simulink model "Engine"  (Simulink 9.3)
settings: Solver=ode23tb  StartTime=0.0  StopTime=50  FixedStep=0.001  EnableMultiTasking=on
values from neighbouring files (symbols this model uses):
  toggle_paf = toggle(2)    [RunEngine.m]
  toggle_vol = toggle(3)    [RunEngine.m]
  toggle_Waf = toggle(4)    [RunEngine.m]
  toggle_Wc = toggle(5)    [RunEngine.m]
  toggle_Wic = toggle(6)    [RunEngine.m]
  toggle_Wth = toggle(7)    [RunEngine.m]
  toggle_xth = toggle(8)    [RunEngine.m]
  toggle_ypic = toggle(9)    [RunEngine.m]
  toggle_ypim = toggle(10)    [RunEngine.m]
  toggle_yTic = toggle(11)    [RunEngine.m]
  toggle_yWaf = toggle(12)    [RunEngine.m]
undefined symbols (not defined in the file or in its folder): a0, a1, a2, dP_thrREF, KpThr, KpWg, n_r, Newton, r_c, Raphson, T_z, TC_ENGINE, TiThr, TiWg
libraries: simulink x3
(part 1 of 3)
settings Model: Creator=Mark Ng  LastModifiedBy=markng  ExtModeTrigMode=oneshot  ExtModeArmWhenConnect=off  ExtModeAutoUpdateStatusClock=off
settings SolverCC: MaxConsecutiveMinStep=100  ZeroCrossControl=EnableAll  SolverResetMethod=Robust
settings DataIOCC: SignalLoggingName=sigsOut
settings OptimizationCC: BooleanDataType=off  ExpressionDepthLimit=2147483647  InitFltsAndDblsToZero=on  SimCompilerOptimization=on
settings DebuggingCC: SaveWithParameterizedLinksMsg=none  SignalResolutionControl=TryResolveAllWithWarning  MaxConsecutiveZCsMsg=none  MultiTaskDSMMsg=warning  MultiTaskCondExecSysMsg=none  StateNameClashWarn=warning  PregeneratedLibrarySubsystemCodeDiagnostic=none
settings HardwareCC: TargetBitPerLong=64  TargetBitPerPointer=64  TargetBitPerSizeT=64  TargetBitPerPtrDiffT=64  TargetLongLongMode=on  TargetIntDivRoundTo=Zero  TargetEndianess=LittleEndian  TargetWordSize=64  TargetHWDeviceType=MATLAB Host  ProdEqTarget=off
settings GRTTargetCC: TargetFcnLib=ansi_tfl_tmw.mat  CompOptLevelCompliant=off  GeneratePreprocessorConditionals=Disable all

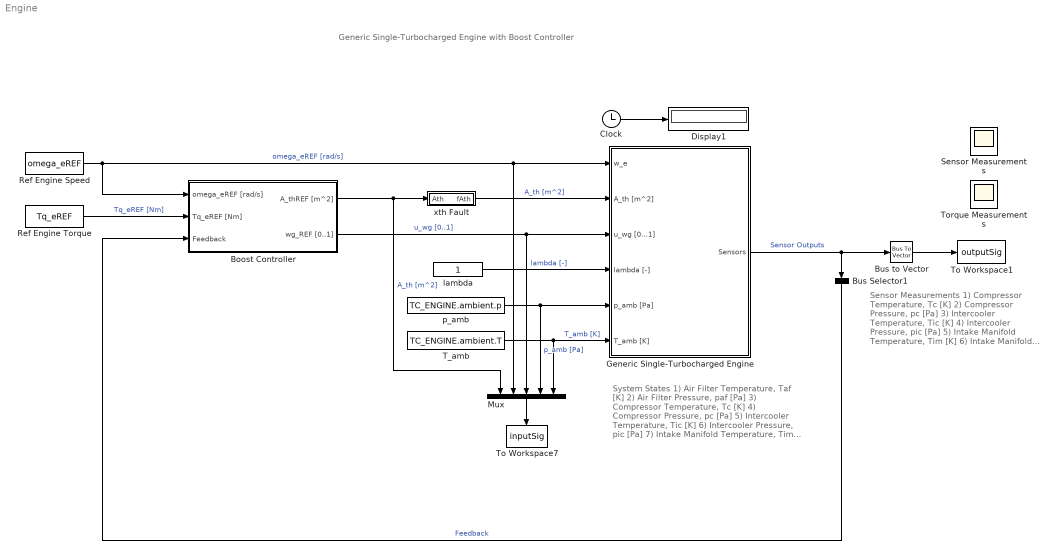
== system Engine ==
  note: Sensor Measurements
      |
      | 1) Compressor Temperature, Tc [K]
      | 2) Compressor Pressure, pc [Pa]
      | 3) Intercooler Temperature, Tic [K]
      | 4) Intercooler Pressure, pic [Pa]
      | 5) Intake Manifold Temperature, Tim [K]
      | 6) Intake Manifold Pressure, pim [Pa]
      | 7) Air Filter Mass Flow, Waf [kg/s]
      | 8) Engine Torque, Tq_e [Nm]
      | 9) Exhaust Manifold Pressure, pem [Pa]
  note: System States
      |
      |   1) Air Filter Temperature, Taf [K]
      |   2) Air Filter Pressure, paf [Pa]
      |   3) Compressor Temperature, Tc [K]
      |   4) Compressor Pressure, pc [Pa]
      |   5) Intercooler Temperature, Tic [K]
      |   6) Intercooler Pressure, pic [Pa]
      |   7) Intake Manifold Temperature, Tim [K]
      |   8) Intake Manifold Pressure, pim [Pa]
      |   9) Exhaust Manifold Temperature, Tem [K]
      | 10) Exhaust Manifold Pressure, pem [Pa]
      | 11) Turbine Temperature, Tt [K]
      | 12) Turbine Pressure, pt [Pa]
      | 13) Turbine Speed, omega_t [rad/s]
  note: Generic Single-Turbocharged Engine
      | with Boost Controller
  Boost Controller : Subsystem
  Bus Selector1 : BusSelector  OutputSignals=p_ic [Pa],p_im [Pa],T_im [K],p_em [Pa],Tq_e [Nm]  OutputAsBus=on
  Bus to Vector : BusToVector
  Clock : Clock
  Display1 : Display
  Generic Single-Turbocharged Engine : Subsystem
  Mux : Mux  Inputs=5
  Ref Engine Speed : FromWorkspace  VariableName=omega_eREF  SampleTime=0
  Ref Engine Torque : FromWorkspace  VariableName=Tq_eREF  SampleTime=0
  Sensor Measurements : Scope
      settings: Floating=on
  T_amb : Constant  Value=TC_ENGINE.ambient.T
  To Workspace1 : ToWorkspace  VariableName=outputSig  SaveFormat=Timeseries  SampleTime=-1
  To Workspace7 : ToWorkspace  VariableName=inputSig  SaveFormat=Timeseries  SampleTime=-1
  Torque Measurements : Scope
      settings: Floating=on
  lambda : Constant
  p_amb : Constant  Value=TC_ENGINE.ambient.p
  xth Fault : Subsystem
  wires:
  Clock/1 -> Display1/1
  lambda/1 -> Generic Single-Turbocharged Engine/4(lambda [-])  "lambda [-]"
  T_amb/1 -> Mux/5, Generic Single-Turbocharged Engine/6(T_amb [K])  "T_amb [K]"
  Boost Controller/1(A_thREF [m^2]) -> xth Fault/1(Ath), Mux/1  "A_th [m^2]"
  p_amb/1 -> Mux/4, Generic Single-Turbocharged Engine/5(p_amb [Pa])  "p_amb [Pa]"
  Boost Controller/2(wg_REF [0..1]) -> Mux/3, Generic Single-Turbocharged Engine/3(u_wg [0...1])  "u_wg [0..1]"
  xth Fault/1(fAth) -> Generic Single-Turbocharged Engine/2(A_th [m^2])  "A_th [m^2]"
  Ref Engine Torque/1 -> Boost Controller/2(Tq_eREF [Nm])  "Tq_eREF [Nm]"
  Ref Engine Speed/1 -> Mux/2, Generic Single-Turbocharged Engine/1(w_e), Boost Controller/1("omega_eREF [rad/s] ")  "omega_eREF [rad/s]"
  Bus Selector1/1 -> Boost Controller/3(Feedback)  "Feedback"
  Generic Single-Turbocharged Engine/1(Sensors) -> Bus to Vector/1, Bus Selector1/1  "Sensor Outputs"
  Mux/1 -> To Workspace7/1
  Bus to Vector/1 -> To Workspace1/1

== system Engine/Boost Controller ==
  "omega_eREF [rad/s] " : Inport
  Tq_eREF [Nm] : Inport  Port=2
  Feedback : Inport  Port=3
  Bus Selector : BusSelector  OutputSignals=Tq_e [Nm],T_im [K],p_em [Pa],p_ic [Pa],p_im [Pa]
  Driver gas pedal interpretation : Subsystem
  Subsystem : Subsystem
  Subtract1 : Sum
  Throttle saturation [0..1] : Saturate  UpperLimit=1  LowerLimit=0
  "Throttle Feed Forward " : Subsystem
  Throttle Feedback including anti-windup : Subsystem
  Waste-gate saturation [0..1] : Saturate  UpperLimit=1  LowerLimit=0
  Waste-gate Feedback including anti-windup : Subsystem
  A_thREF [m^2] : Outport
  wg_REF [0..1] : Outport  Port=2
  wires:
  "omega_eREF [rad/s] "/1 -> "Throttle Feed Forward "/2(N_e [rad/s])
  Throttle saturation [0..1]/1 -> Subsystem/1(In1), Throttle Feedback including anti-windup/3(alpha_thrREFsat [0..1])
  Waste-gate saturation [0..1]/1 -> Waste-gate Feedback including anti-windup/3(wgREFsat [0..1]), wg_REF [0..1]/1
  Bus Selector/4 -> Waste-gate Feedback including anti-windup/2(p_icACT [Pa]), "Throttle Feed Forward "/3(p_icACT [Pa])  "<p_ic [Pa]>"
  Bus Selector/5 -> Throttle Feedback including anti-windup/2(p_imACT [Pa]), Driver gas pedal interpretation/3(p_im [Pa])  "<p_im [Pa]>"
  Driver gas pedal interpretation/1(p_im_ref) -> Throttle Feedback including anti-windup/1(p_imREF [Pa]), "Throttle Feed Forward "/1(p_imREF [Pa])
  Driver gas pedal interpretation/2(p_ic_ref) -> Waste-gate Feedback including anti-windup/1(p_icREF [Pa])
  Tq_eREF [Nm]/1 -> Driver gas pedal interpretation/1(Tq_eREF [Nm])
  Subsystem/1(Out1) -> A_thREF [m^2]/1
  Bus Selector/1 -> Driver gas pedal interpretation/2(Tq_e [Nm])  "<Tq_e [Nm]>"
  Bus Selector/2 -> "Throttle Feed Forward "/4(T_im [K])  "<T_im [K]>"
  Bus Selector/3 -> "Throttle Feed Forward "/5("p_em ")  "<p_em [Pa]>"
  Throttle Feedback including anti-windup/1(alpha_thrFB [0..1]) -> Subtract1/2
  "Throttle Feed Forward "/1(alpha_thrFF [0..1]) -> Subtract1/1
  Subtract1/1 -> Throttle saturation [0..1]/1, Throttle Feedback including anti-windup/4(alpha_thrREF [0..1])
  Waste-gate Feedback including anti-windup/1(wgFB [0..1]) -> Waste-gate saturation [0..1]/1, Waste-gate Feedback including anti-windup/4(wgREF [0..1])
  Feedback/1 -> Bus Selector/1

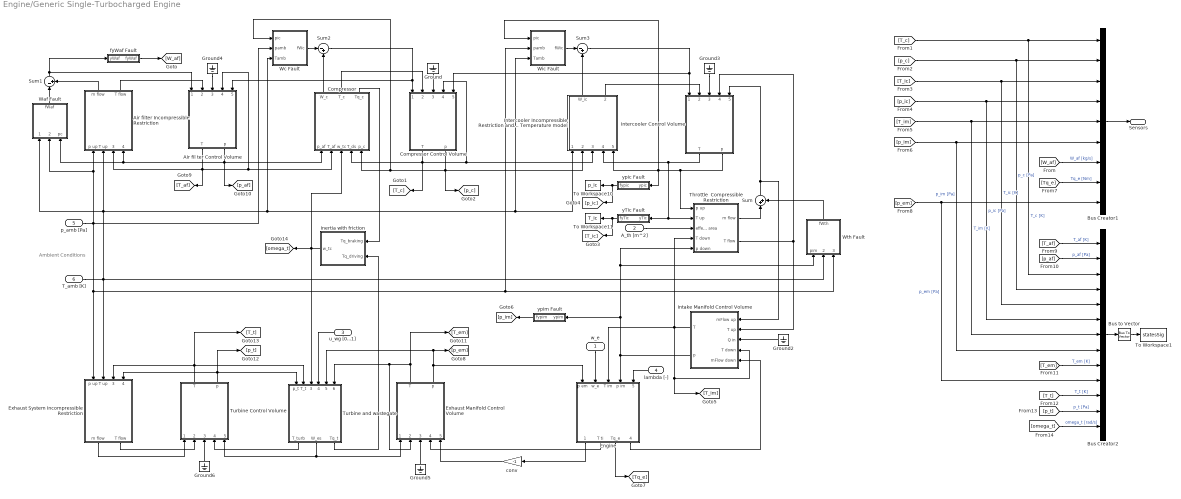
== system Engine/Generic Single-Turbocharged Engine ==
  note: Ambient Conditions
  w_e : Inport
  A_th [m^2] : Inport  Port=2
  u_wg [0...1] : Inport  Port=3
  lambda [-] : Inport  Port=4
  p_amb [Pa] : Inport  Port=5
  T_amb [K] : Inport  Port=6
  Air fil ter Control Volume : Subsystem  mask(Control volume){V=TC_ENGINE.controlVolumes.airFilter.V, T_init=293, p_init=101e3, R=TC_ENGINE.gasProp.air.R, gamma=TC_ENGINE.gasProp.air.kappa}
      mask prompts: V "Volume [m^3]"; T_init "Initial temperature [K]"; p_init "Initial pressure [Pa]"; R "Gas constant [J/kg K]"; gamma "Ratio of specific heats (gamma) [-]"
      mask help:
      | Model of a control volume i.e. a receiver of constant volume.
      | Takes mass and energy balance into account.
      | <br>
      | m'=m_in-m_out
      | <br>
      | T'=(H_in - H_out - Q_out - m' c_v) / m / c_v
      mask Help:
      | Models a receiver of constant volume.
      | Takes mass and energy balance into account.
      | m_in    - mass flow in
      | m_out - mass flow out
      | m'=m_in-m_out
      | T'=(m_in c_v (T_i-T)+ R (T_i m_in -T m_out)+Q_in)/m/c_v
  Air filter Incompressible Restriction : Subsystem  mask(Restriction Incompressible Flow){H=TC_ENGINE.airFilter.H, p_lin=TC_ENGINE.airFilter.p_lin}
      mask prompts: H "Flow resistance"; p_lin "Linearization limit [Pa]"
      mask help:
      | Flow restriction for incompressible flows.
      |
      | The flow is modelled using the following function for the pressure drop over the system where the conditions refer to upstream conditions.
      |
      | delta p=H mFlow^2 T_in/p_in
      mask Help:
      | <h3>Flow restriction for incompressible flows.</h3>
      | <br>
      | The flow is modelled using the following function for the pressure drop over the system where the conditions refer to upstream conditions.
      | <br>
      | delta p=H mFlow^2 T_in/p_in
  Bus Creator1 : BusCreator  Inputs=9
  Bus Creator2 : BusCreator  Inputs=13
  Bus to Vector : BusToVector
  Compressor : Subsystem
  Compressor Control Volume : Subsystem  mask(Control volume){V=TC_ENGINE.controlVolumes.compressor.V, T_init=293, p_init=101e3, R=TC_ENGINE.gasProp.air.R, gamma=TC_ENGINE.gasProp.air.kappa}
      mask prompts: V "Volume [m^3]"; T_init "Initial temperature [K]"; p_init "Initial pressure [Pa]"; R "Gas constant [J/kg K]"; gamma "Ratio of specific heats (gamma) [-]"
      mask help:
      | Model of a control volume i.e. a receiver of constant volume.
      | Takes mass and energy balance into account.
      | <br>
      | m'=m_in-m_out
      | <br>
      | T'=(H_in - H_out - Q_out - m' c_v) / m / c_v
      mask Help:
      | Models a receiver of constant volume.
      | Takes mass and energy balance into account.
      | m_in    - mass flow in
      | m_out - mass flow out
      | m'=m_in-m_out
      | T'=(m_in c_v (T_i-T)+ R (T_i m_in -T m_out)+Q_in)/m/c_v
  Engine : Subsystem
  Exhaust Manifold Control Volume : Subsystem  mask(Control volume){V=TC_ENGINE.controlVolumes.exhaustManifold.V, T_init=900, p_init=105e3, R=TC_ENGINE.gasProp.exh.R, gamma=TC_ENGINE.gasProp.exh.kappa}
      mask prompts: V "Volume [m^3]"; T_init "Initial temperature [K]"; p_init "Initial pressure [Pa]"; R "Gas constant [J/kg K]"; gamma "Ratio of specific heats (gamma) [-]"
      mask help:
      | Model of a control volume i.e. a receiver of constant volume.
      | Takes mass and energy balance into account.
      | <br>
      | m'=m_in-m_out
      | <br>
      | T'=(H_in - H_out - Q_out - m' c_v) / m / c_v
      mask Help:
      | Models a receiver of constant volume.
      | Takes mass and energy balance into account.
      | m_in    - mass flow in
      | m_out - mass flow out
      | m'=m_in-m_out
      | T'=(m_in c_v (T_i-T)+ R (T_i m_in -T m_out)+Q_in)/m/c_v
  Exhaust System Incompressible Restriction : Subsystem  mask(Restriction Incompressible Flow){H=TC_ENGINE.exhaustSystem.H, p_lin=TC_ENGINE.exhaustSystem.p_lin}
      mask prompts: H "Flow resistance"; p_lin "Linearization limit [Pa]"
      mask help:
      | Flow restriction for incompressible flows.
      |
      | The flow is modelled using the following function for the pressure drop over the system where the conditions refer to upstream conditions.
      |
      | delta p=H mFlow^2 T_in/p_in
      mask Help:
      | <h3>Flow restriction for incompressible flows.</h3>
      | <br>
      | The flow is modelled using the following function for the pressure drop over the system where the conditions refer to upstream conditions.
      | <br>
      | delta p=H mFlow^2 T_in/p_in
  Ground{,2..6} (6 alike) : Ground
  Inertia with friction : Subsystem  mask(Inertia with friction){Theta=TC_ENGINE.turbo.inertia_tc, w_friction=TC_ENGINE.turbo.damp_tc, w_IC=TC_ENGINE.turbo.omega_init, w_upper=TC_ENGINE.turbo.omega_max, w_lower=TC_ENGINE.turbo.omega_min}
      mask prompts: Theta "Inertia [kg m^2]"; w_friction "Friction coefficient"; w_IC "Initial rotational speed [rad/s]"; w_upper "Upper speed limit [rad/s]"; w_lower "Lower speed limit [rad/s]"
      mask help:
      | Rotating inertia, with inputs speed. There is also a friction term which might help stabilize the simulated system for some conditions.
      |
      | Additionally it is possible to have upper and lower limits on the speed.
      mask Help:
      | Rotating inertia, with inputs speed. There is also a friction term which might help stabilize the simulated system for some conditions.
      | 
      | <br>
      | 
      | Additionally it is possible to have upper and lower limits on the speed.
  Intake Manifold Control Volume : Subsystem  mask(Control volume){V=TC_ENGINE.controlVolumes.intakeManifold.V, T_init=293, p_init=101e3, R=TC_ENGINE.gasProp.air.R, gamma=TC_ENGINE.gasProp.air.kappa}
      mask prompts: V "Volume [m^3]"; T_init "Initial temperature [K]"; p_init "Initial pressure [Pa]"; R "Gas constant [J/kg K]"; gamma "Ratio of specific heats (gamma) [-]"
      mask help:
      | Model of a control volume i.e. a receiver of constant volume.
      | Takes mass and energy balance into account.
      | <br>
      | m'=m_in-m_out
      | <br>
      | T'=(H_in - H_out - Q_out - m' c_v) / m / c_v
      mask Help:
      | Models a receiver of constant volume.
      | Takes mass and energy balance into account.
      | m_in    - mass flow in
      | m_out - mass flow out
      | m'=m_in-m_out
      | T'=(m_in c_v (T_i-T)+ R (T_i m_in -T m_out)+Q_in)/m/c_v
  Intercooler Control Volume : Subsystem  mask(Control volume){V=TC_ENGINE.controlVolumes.interCooler.V, T_init=293, p_init=101e3, R=TC_ENGINE.gasProp.air.R, gamma=TC_ENGINE.gasProp.air.kappa}
      mask prompts: V "Volume [m^3]"; T_init "Initial temperature [K]"; p_init "Initial pressure [Pa]"; R "Gas constant [J/kg K]"; gamma "Ratio of specific heats (gamma) [-]"
      mask help:
      | Model of a control volume i.e. a receiver of constant volume.
      | Takes mass and energy balance into account.
      | <br>
      | m'=m_in-m_out
      | <br>
      | T'=(H_in - H_out - Q_out - m' c_v) / m / c_v
      mask Help:
      | Models a receiver of constant volume.
      | Takes mass and energy balance into account.
      | m_in    - mass flow in
      | m_out - mass flow out
      | m'=m_in-m_out
      | T'=(m_in c_v (T_i-T)+ R (T_i m_in -T m_out)+Q_in)/m/c_v
  Intercooler Incompressible Restriction and Temperature model : Subsystem
  Sum : Sum  Inputs=|++
  Sum1 : Sum  Inputs=|-+
  Sum2 : Sum  Inputs=|-+
  Sum3 : Sum  Inputs=|-+
  Throttle  Compressible Restriction : Subsystem  mask(Restriction - Compressible Flow){K=TC_ENGINE.throttle.gamma, R=TC_ENGINE.gasProp.air.R}
      mask prompts: K "Ratio of specific heats"; R "Ideal gas constant [J/kg/ K]"
      mask help:
      | The flow is modelled using isentropic expansion in a nozzle with the assumption that there is no pressure recovery after the nozzle.
      |
      | See e.g. Heywood Appendix C for a derivation.
      mask Help:
      | <h3>Flow restriction for compressible flows.</h3>
      | <br>
      | The flow is modelled using isentropic expansion in a nozzle with the assumption that there is no pressure recovery after the nozzle.
      | 
      | See e.g. Heywood Appendix C for a derivation.
  To Workspace1 : ToWorkspace  VariableName=statesSig  SaveFormat=Timeseries  SampleTime=-1
  To Workspace10 : ToWorkspace  VariableName=p_ic  SaveFormat=Timeseries  SampleTime=-1
  To Workspace11 : ToWorkspace  VariableName=T_ic  SaveFormat=Timeseries  SampleTime=-1
  Turbine Control Volume : Subsystem  mask(Control volume){V=TC_ENGINE.controlVolumes.exhaustSystem.V, T_init=293, p_init=101e3, R=TC_ENGINE.gasProp.exh.R, gamma=TC_ENGINE.gasProp.exh.kappa}
      mask prompts: V "Volume [m^3]"; T_init "Initial temperature [K]"; p_init "Initial pressure [Pa]"; R "Gas constant [J/kg K]"; gamma "Ratio of specific heats (gamma) [-]"
      mask help:
      | Model of a control volume i.e. a receiver of constant volume.
      | Takes mass and energy balance into account.
      | <br>
      | m'=m_in-m_out
      | <br>
      | T'=(H_in - H_out - Q_out - m' c_v) / m / c_v
      mask Help:
      | Models a receiver of constant volume.
      | Takes mass and energy balance into account.
      | m_in    - mass flow in
      | m_out - mass flow out
      | m'=m_in-m_out
      | T'=(m_in c_v (T_i-T)+ R (T_i m_in -T m_out)+Q_in)/m/c_v
  Turbine and wastegate : Subsystem
  Waf Fault : Subsystem  mask{K=TC_ENGINE.gasProp.air.kappa}
      mask prompts: K "Ratio of throttle specific heat"
  Wc Fault : Subsystem  mask{K=TC_ENGINE.gasProp.air.kappa}
      mask prompts: K "Ratio of throttle specific heat"
  Wic Fault : Subsystem  mask{K=TC_ENGINE.gasProp.air.kappa}
      mask prompts: K "Ratio of throttle specific heat"
  Wth Fault : Subsystem  mask{K=TC_ENGINE.throttle.gamma}
      mask prompts: K "Ratio of throttle specific heat"
  conv : Gain  Gain=-1  SaturateOnIntegerOverflow=on  OutDataTypeStr=Inherit: Same as input  ParamDataTypeStr=Inherit: Same as input
  fyWaf Fault : Subsystem
  yTic Fault : Subsystem
  ypic Fault : Subsystem
  ypim Fault : Subsystem
  Sensors : Outport
  wires:
  T_amb [K]/1 -> Air filter Incompressible Restriction/2(T up), Wic Fault/3(Tamb), Intercooler Incompressible Restriction and Temperature model/1(T_cool [K]), Wc Fault/3(Tamb), Waf Fault/1(Tamb), Wth Fault/2(Tamb), Exhaust System Incompressible Restriction/2(T up)
  Air fil ter Control Volume/1(T) -> [T_af], Air filter Incompressible Restriction/3(T down), Compressor/2(T_af), Air fil ter Control Volume/4(T down)
  Ground4/1 -> Air fil ter Control Volume/3(Q in)
  Air filter Incompressible Restriction/2(T flow) -> Air fil ter Control Volume/2(T up)
  p_amb [Pa]/1 -> Wth Fault/3(pamb), Wic Fault/2(pamb), Exhaust System Incompressible Restriction/1(p up), Waf Fault/2(pamb), Air filter Incompressible Restriction/1(p up), Wc Fault/2(pamb)
  Compressor Control Volume/1(T) -> Compressor Control Volume/4(T down), Intercooler Incompressible Restriction and Temperature model/3(T_up), [T_c], Compressor/4(T_ds)
  Ground/1 -> Compressor Control Volume/3(Q in)
  Sum2/1 -> Compressor Control Volume/1(mFlow up), Air fil ter Control Volume/5(mFlow down)
  Sum/1 -> Intake Manifold Control Volume/1(mFlow up), Intercooler Control Volume/5(mFlow down)
  Throttle  Compressible Restriction/2(T flow) -> Intake Manifold Control Volume/2(T up), Intercooler Control Volume/4(T down)
  Ground2/1 -> Intake Manifold Control Volume/3(Q in)
  Intake Manifold Control Volume/1(T) -> Throttle  Compressible Restriction/4(T down), Engine/3(T im), [T_im], Intake Manifold Control Volume/4(T down)
  A_th [m^2]/1 -> Throttle  Compressible Restriction/3(effective area)
  w_e/1 -> Engine/2(w_e)
  Engine/4(air Flow) -> Intake Manifold Control Volume/5(mFlow down)
  Engine/1(mFlow e) -> conv/1
  Ground3/1 -> Intercooler Control Volume/3(Q in)
  conv/1 -> Exhaust Manifold Control Volume/5(mFlow down)
  Engine/2(T ti) -> Exhaust Manifold Control Volume/4(T down)
  Ground5/1 -> Exhaust Manifold Control Volume/3(Q in)
  Exhaust Manifold Control Volume/2(p) -> Engine/1(p em), [p_em], Turbine and wastegate/5(p_em)
  Turbine Control Volume/1(T) -> [T_t], Exhaust System Incompressible Restriction/3(T down), Turbine and wastegate/2(T_t)
  Turbine Control Volume/2(p) -> [p_t], Turbine and wastegate/1(p_t), Exhaust System Incompressible Restriction/4(p down)
  Turbine and wastegate/1(T_turb) -> Turbine Control Volume/4(T down)
  Ground6/1 -> Turbine Control Volume/3(Q in)
  Exhaust System Incompressible Restriction/2(T flow) -> Turbine Control Volume/2(T up)
  Exhaust System Incompressible Restriction/1(m flow) -> Turbine Control Volume/1(mFlow up)
  lambda [-]/1 -> Engine/5(lambda)
  Compressor Control Volume/2(p) -> [p_c], Intercooler Incompressible Restriction and Temperature model/2(p_up), Compressor/5(p_c), Wc Fault/1("pic ")
  Intercooler Incompressible Restriction and Temperature model/2(T_fwd_flow [K]) -> Intercooler Control Volume/2(T up)
  Intercooler Control Volume/1(T) -> Intercooler Incompressible Restriction and Temperature model/4(T_down), yTic Fault/1(yTic), Throttle  Compressible Restriction/2(T up)
  Compressor/2(T_c) -> Compressor Control Volume/2(T up)
  Sum3/1 -> Compressor Control Volume/5(mFlow down), Intercooler Control Volume/1(mFlow up)
  fyWaf Fault/1(fyWaf) -> [W_af]
  Compressor/3(Tq_c) -> Inertia with friction/1(Tq_braking)
  u_wg [0...1]/1 -> Turbine and wastegate/4(u_wg)
  Exhaust Manifold Control Volume/1(T) -> [T_em], Exhaust Manifold Control Volume/2(T up), Turbine and wastegate/6(T_em)
  Turbine and wastegate/3(Tq_t) -> Inertia with friction/2(Tq_driving)
  Turbine and wastegate/2(W_es) -> Exhaust Manifold Control Volume/1(mFlow up), Turbine Control Volume/5(mFlow down)
  yTic Fault/1(fyTic) -> [T_ic], To Workspace11/1
  ypic Fault/1(fypic) -> [p_ic], To Workspace10/1
  Throttle  Compressible Restriction/1(m flow) -> Sum/1
  Wth Fault/1(fWth) -> Sum/2
  ypim Fault/1(fypim) -> [p_im]
  Waf Fault/1(fWaf) -> Sum1/1
  Air filter Incompressible Restriction/1(m flow) -> Sum1/2
  Sum1/1 -> fyWaf Fault/1(yWaf), Air fil ter Control Volume/1(mFlow up)
  Wc Fault/1(fWc) -> Sum2/1
  Compressor/1(W_c) -> Sum2/2
  Intercooler Control Volume/2(p) -> Intercooler Incompressible Restriction and Temperature model/5(p_down), Wic Fault/1("pic "), ypic Fault/1(ypic), Throttle  Compressible Restriction/1(p up)
  Wic Fault/1(fWic) -> Sum3/1
  Intercooler Incompressible Restriction and Temperature model/1(W_ic) -> Sum3/2
  Intake Manifold Control Volume/2(p) -> ypim Fault/1(ypim), Throttle  Compressible Restriction/5(p down), Wth Fault/1(pim), Engine/4(p im)
  Engine/3(Tq_e) -> [Tq_e]
  [T_ic] -> Bus Creator2/5, Bus Creator1/3  "T_ic [K]"
  [T_c] -> Bus Creator1/1, Bus Creator2/3  "T_c [K]"
  [p_c] -> Bus Creator2/4, Bus Creator1/2  "p_c [Pa]"
  [T_im] -> Bus Creator1/5, Bus Creator2/7  "T_im [K]"
  [W_af] -> Bus Creator1/7  "W_af [kg/s]"
  [Tq_e] -> Bus Creator1/8  "Tq_e [Nm]"
  [p_im] -> Bus Creator2/8, Bus Creator1/6  "p_im [Pa]"
  [p_ic] -> Bus Creator2/6, Bus Creator1/4  "p_ic [Pa]"
  [p_em] -> Bus Creator2/10, Bus Creator1/9  "p_em [Pa]"
  Bus Creator1/1 -> Sensors/1
  Bus Creator2/1 -> Bus to Vector/1
  [T_af] -> Bus Creator2/1  "T_af [K]"
  Air fil ter Control Volume/2(p) -> [p_af], Waf Fault/3("pc "), Air filter Incompressible Restriction/4(p down), Compressor/1(p_af)
  [p_af] -> Bus Creator2/2  "p_af [Pa]"
  [T_em] -> Bus Creator2/9  "T_em [K]"
  [T_t] -> Bus Creator2/11  "T_t [K]"
  [p_t] -> Bus Creator2/12  "p_t [Pa]"
  [omega_t] -> Bus Creator2/13  "omega_t [rad/s]"
  Inertia with friction/1(w_tc) -> [omega_t], Turbine and wastegate/3(w_tc), Compressor/3(w_tc)
  Bus to Vector/1 -> To Workspace1/1

== system Engine/xth Fault ==
  Ath : Inport
  Step : Step  Time=0.4*size(T_z,1)  SampleTime=0
  Sum : Sum  Inputs=|++
  To Workspace2 : ToWorkspace  VariableName=fxthSig  SaveFormat=Timeseries  SampleTime=-1
  "toggle " : Gain  Gain=toggle_xth*0.5e-6  SaturateOnIntegerOverflow=on  OutDataTypeStr=Inherit: Same as input  ParamDataTypeStr=Inherit: Same as input
  fAth : Outport
  wires:
  Ath/1 -> Sum/1
  Sum/1 -> fAth/1
  "toggle "/1 -> To Workspace2/1, Sum/2
  Step/1 -> "toggle "/1

== system Engine/Boost Controller/Driver gas pedal interpretation ==
  note: Cp1
  note: Cp0
  Tq_eREF [Nm] : Inport
  Tq_e [Nm] : Inport  Port=2
  p_im [Pa] : Inport  Port=3
  Add2 : Sum
  Add3 : Sum
  Demux : Demux  Outputs=2
  Divide : Product  Inputs=*/
  Gain : Gain  Gain=2*pi*n_r/TC_ENGINE.geometry.V_d
  Interpreted MATLAB Function : MATLABFcn  MATLABFcn=pinv([-1 u(1)])
  Product : Product
  To Workspace1 : ToWorkspace  VariableName=p_ic_REF  SaveFormat=Timeseries  SampleTime=-1
  To Workspace6 : ToWorkspace  VariableName=p_im_REF  SaveFormat=Timeseries  SampleTime=-1
  Tq2BMEP : Gain  Gain=2*pi*n_r/TC_ENGINE.geometry.V_d
  a0 : Constant  Value=dP_thrREF
  p_im_ref : Outport
  p_ic_ref : Outport  Port=2
  wires:
  Tq2BMEP/1 -> Add2/1  "BMEP_REF"
  Demux/1 -> Add2/2
  Add2/1 -> Divide/1
  Demux/2 -> Divide/2
  Divide/1 -> Add3/1, To Workspace6/1, p_im_ref/1  "p_im_REF"
  Add3/1 -> To Workspace1/1, p_ic_ref/1  "p_ic_REF"
  a0/1 -> Add3/2
  Tq_eREF [Nm]/1 -> Tq2BMEP/1
  p_im [Pa]/1 -> Interpreted MATLAB Function/1
  Interpreted MATLAB Function/1 -> Product/1
  Tq_e [Nm]/1 -> Gain/1
  Gain/1 -> Product/2
  Product/1 -> Demux/1

== system Engine/Boost Controller/Subsystem ==
  In1 : Inport
  "% -> Area" : Subsystem
  mm2->m^2 : Gain  Gain=1e-6  SaturateOnIntegerOverflow=on  OutDataTypeStr=Inherit: Same as input  ParamDataTypeStr=Inherit: Same as input
  Out1 : Outport
  wires:
  In1/1 -> "% -> Area"/1(%)
  "% -> Area"/1(A) -> mm2->m^2/1
  mm2->m^2/1 -> Out1/1

== system Engine/Boost Controller/Throttle Feed Forward  ==
  p_imREF [Pa] : Inport
  N_e [rad/s] : Inport  Port=2
  p_icACT [Pa] : Inport  Port=3
  T_im [K] : Inport  Port=4
  "p_em " : Inport  Port=5
  Aeff2alpha : Subsystem
  Cylinder air flow REF : Subsystem
  Divide : Product  Inputs=*/
  Divide1 : Product  Inputs=*//*
  Max : MinMax  Function=max  Inputs=2
  Product2 : Product  RndMeth=Zero
  Psi(PI) : Subsystem
  R : Constant  Value=TC_ENGINE.gasProp.air.R
  Sqrt : Sqrt  AlgorithmType=Newton-Raphson  SaturateOnIntegerOverflow=on
  Tamb : Constant  Value=TC_ENGINE.ambient.T
  alpha_thrFF [0..1] : Outport
  wires:
  p_imREF [Pa]/1 -> Max/1, Divide/1, Cylinder air flow REF/1(p_im_REF)
  p_icACT [Pa]/1 -> Max/2, Divide1/3
  Cylinder air flow REF/1(m_dot_ac_REF) -> Divide1/1
  Product2/1 -> Sqrt/1  "RT"
  R/1 -> Product2/1  "R"
  Tamb/1 -> Product2/2  "T"
  Divide/1 -> Psi(PI)/1(PI)  "PI_REF"
  Psi(PI)/1(Psi) -> Divide1/2  "Psi_REF"
  Sqrt/1 -> Divide1/4
  Max/1 -> Divide/2
  Aeff2alpha/1(alpha_REF) -> alpha_thrFF [0..1]/1  "alpha_REF"
  Divide1/1 -> Aeff2alpha/1(Aeff_REF)  "Aeff_REF"
  T_im [K]/1 -> Cylinder air flow REF/2(T_im [K])
  N_e [rad/s]/1 -> Cylinder air flow REF/3(N [rad/s])
  "p_em "/1 -> Cylinder air flow REF/4("p_em ")

== system Engine/Boost Controller/Throttle Feedback including anti-windup ==
  p_imREF [Pa] : Inport
  p_imACT [Pa] : Inport  Port=2
  alpha_thrREFsat [0..1] : Inport  Port=3
  alpha_thrREF [0..1] : Inport  Port=4
  Constant : Constant
  Integrator1 : Integrator  UpperSaturationLimit=5  LowerSaturationLimit=-5
  Subtract1 : Sum
  Subtract2 : Sum  Inputs=+-
  Subtract3 : Sum  Inputs=-+
  Subtract4 : Sum
  Sum : Sum  Inputs=|++
  u_FB_wg_Kp : Gain  Gain=KpThr
  u_FB_wg_Kp1 : Gain  Gain=KpThr/TiThr
  u_FB_wg_Kp2 : Gain  Gain=1/TiThr
  alpha_thrFB [0..1] : Outport
  wires:
  p_imACT [Pa]/1 -> Subtract3/1
  p_imREF [Pa]/1 -> Subtract3/2
  Subtract3/1 -> u_FB_wg_Kp/1, u_FB_wg_Kp1/1  "controller error"
  u_FB_wg_Kp/1 -> Subtract4/1
  Subtract4/1 -> alpha_thrFB [0..1]/1
  u_FB_wg_Kp1/1 -> Subtract1/1
  alpha_thrREFsat [0..1]/1 -> Subtract2/1
  alpha_thrREF [0..1]/1 -> Subtract2/2
  Subtract2/1 -> u_FB_wg_Kp2/1
  u_FB_wg_Kp2/1 -> Subtract1/2
  Integrator1/1 -> Subtract4/2
  Constant/1 -> Sum/2
  Subtract1/1 -> Sum/1
  Sum/1 -> Integrator1/1

== system Engine/Boost Controller/Waste-gate Feedback including anti-windup ==
  p_icREF [Pa] : Inport
  p_icACT [Pa] : Inport  Port=2
  wgREFsat [0..1] : Inport  Port=3
  wgREF [0..1] : Inport  Port=4
  Integrator1 : Integrator  InitialCondition=0.1
  Subtract1 : Sum
  Subtract2 : Sum  Inputs=+-
  Subtract3 : Sum  Inputs=+-
  Subtract4 : Sum
  Tracking : Gain  Gain=1/TiWg
  u_FB_wg_Integral : Gain  Gain=KpWg/TiWg
  u_FB_wg_Proportional : Gain  Gain=KpWg
  wgFB [0..1] : Outport
  wires:
  Integrator1/1 -> Subtract4/2
  Subtract1/1 -> Integrator1/1
  Tracking/1 -> Subtract1/2
  Subtract2/1 -> Tracking/1
  wgREF [0..1]/1 -> Subtract2/2
  wgREFsat [0..1]/1 -> Subtract2/1
  u_FB_wg_Integral/1 -> Subtract1/1
  Subtract4/1 -> wgFB [0..1]/1
  u_FB_wg_Proportional/1 -> Subtract4/1
  Subtract3/1 -> u_FB_wg_Proportional/1, u_FB_wg_Integral/1  "controller error"
  p_icACT [Pa]/1 -> Subtract3/1
  p_icREF [Pa]/1 -> Subtract3/2

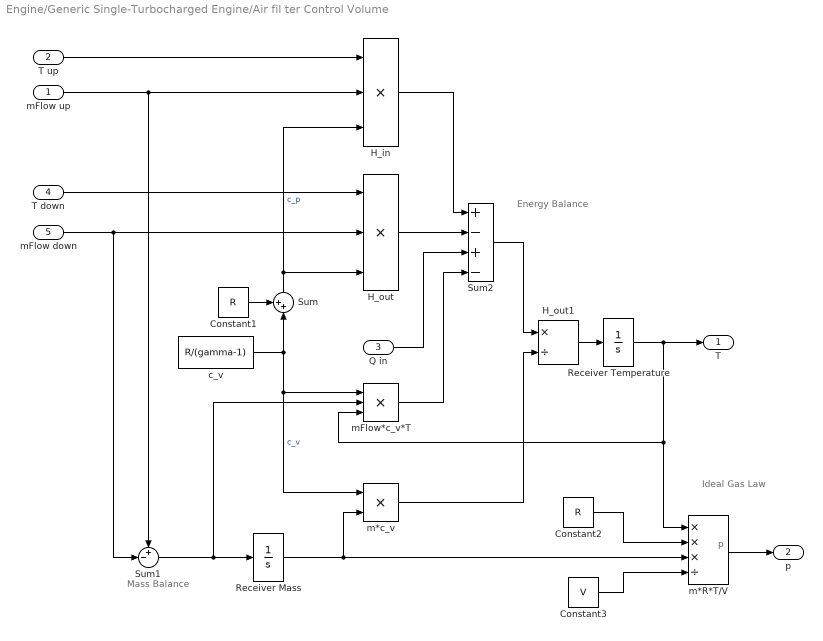
== system Engine/Generic Single-Turbocharged Engine/Air fil ter Control Volume ==
  note: Ideal Gas
      | Law
  note: Energy
      | Balance
  note: Mass
      | Balance
  note: p
  mFlow up : Inport
  T up : Inport  Port=2
  Q in : Inport  Port=3
  T down : Inport  Port=4
  mFlow down : Inport  Port=5
  Constant1 : Constant  Value=R
  Constant2 : Constant  Value=R
  Constant3 : Constant  Value=V
  H_in : Product  Inputs=3  SaturateOnIntegerOverflow=on  InputSameDT=on  OutDataTypeStr=Inherit: Same as first input
  H_out : Product  Inputs=3  SaturateOnIntegerOverflow=on  InputSameDT=on  OutDataTypeStr=Inherit: Same as first input
  H_out1 : Product  Inputs=*/  SaturateOnIntegerOverflow=on  InputSameDT=on  OutDataTypeStr=Inherit: Same as first input
  Receiver Mass : Integrator  InitialCondition=p_init*V/R/T_init  ZeroCross=off
  Receiver Temperature : Integrator  InitialCondition=T_init  ZeroCross=off
  Sum : Sum  Inputs=++|  SaturateOnIntegerOverflow=on  InputSameDT=on  OutDataTypeStr=Inherit: Same as first input
  Sum1 : Sum  Inputs=+-|  SaturateOnIntegerOverflow=on  InputSameDT=on  OutDataTypeStr=Inherit: Same as first input
  Sum2 : Sum  Inputs=+-+-  SaturateOnIntegerOverflow=on  InputSameDT=on  OutDataTypeStr=Inherit: Same as first input
  c_v : Constant  Value=R/(gamma-1)
  m*R*T/V : Product  Inputs=***/  SaturateOnIntegerOverflow=on  InputSameDT=on  OutDataTypeStr=Inherit: Same as first input
  m*c_v : Product  SaturateOnIntegerOverflow=on  InputSameDT=on  OutDataTypeStr=Inherit: Same as first input
  mFlow*c_v*T : Product  Inputs=3  SaturateOnIntegerOverflow=on  InputSameDT=on  OutDataTypeStr=Inherit: Same as first input
  T : Outport
  p : Outport  Port=2
  wires:
  mFlow*c_v*T/1 -> Sum2/4
  c_v/1 -> mFlow*c_v*T/1, m*c_v/1, Sum/2  "c_v"
  Sum1/1 -> mFlow*c_v*T/2, Receiver Mass/1
  Receiver Temperature/1 -> mFlow*c_v*T/3, m*R*T/V/1, T/1
  Constant2/1 -> m*R*T/V/2
  Constant3/1 -> m*R*T/V/4
  H_out1/1 -> Receiver Temperature/1
  m*c_v/1 -> H_out1/2
  Sum2/1 -> H_out1/1
  Q in/1 -> Sum2/3
  H_out/1 -> Sum2/2
  H_in/1 -> Sum2/1
  mFlow up/1 -> Sum1/1, H_in/2
  mFlow down/1 -> H_out/2, Sum1/2
  T down/1 -> H_out/1
  T up/1 -> H_in/1
  Constant1/1 -> Sum/1
  Sum/1 -> H_out/3, H_in/3  "c_p"
  Receiver Mass/1 -> m*R*T/V/3, m*c_v/2
  m*R*T/V/1 -> p/1

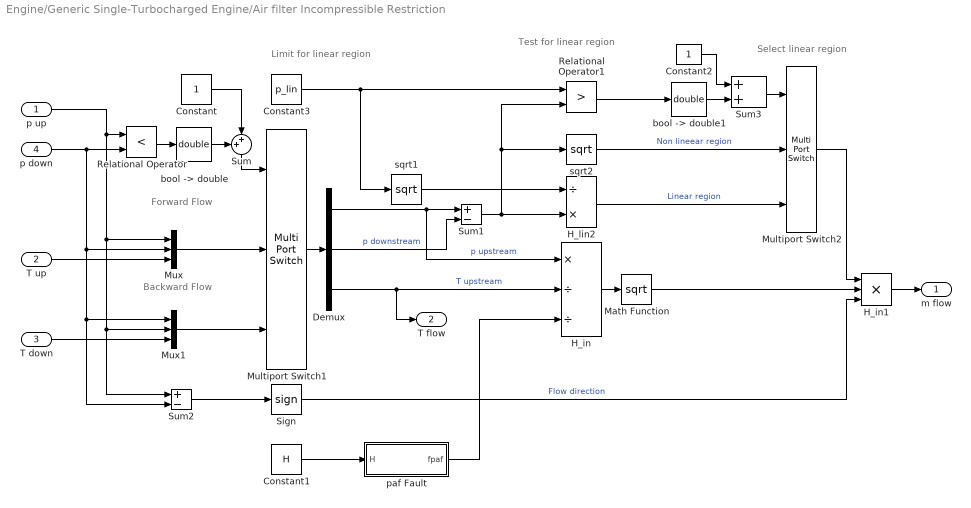
== system Engine/Generic Single-Turbocharged Engine/Air filter Incompressible Restriction ==
  note: Limit for linear region
  note: Select linear region
  note: Test for linear region
  note: Backward
      | Flow
  note: Forward
      | Flow
  p up : Inport
  T up : Inport  Port=2
  T down : Inport  Port=3
  p down : Inport  Port=4
  Constant : Constant
  Constant1 : Constant  Value=H
  Constant2 : Constant
  Constant3 : Constant  Value=p_lin
  Demux : Demux  Outputs=3
  H_in : Product  Inputs=*//  SaturateOnIntegerOverflow=on  InputSameDT=on  OutDataTypeStr=Inherit: Same as first input
  H_in1 : Product  Inputs=3  SaturateOnIntegerOverflow=on  InputSameDT=on  OutDataTypeStr=Inherit: Same as first input
  H_lin2 : Product  Inputs=/*  SaturateOnIntegerOverflow=on  InputSameDT=on  OutDataTypeStr=Inherit: Same as first input
  Math Function : Math  Operator=sqrt  SaturateOnIntegerOverflow=on
  Multiport Switch1 : MultiPortSwitch  Inputs=2  SaturateOnIntegerOverflow=on  InputSameDT=on
  Multiport Switch2 : MultiPortSwitch  Inputs=2  SaturateOnIntegerOverflow=on  InputSameDT=on
  Mux : Mux  Inputs=3
  Mux1 : Mux  Inputs=3
  Relational Operator : RelationalOperator  Operator=<  RndMeth=Nearest  InputSameDT=on
  Relational Operator1 : RelationalOperator  Operator=>  RndMeth=Nearest  InputSameDT=on
  Sign : Signum  ZeroCross=off
  Sum : Sum  Inputs=++|  SaturateOnIntegerOverflow=on  InputSameDT=on  OutDataTypeStr=Inherit: Same as first input
  Sum1 : Sum  Inputs=+-  SaturateOnIntegerOverflow=on  InputSameDT=on  OutDataTypeStr=Inherit: Same as first input
  Sum2 : Sum  Inputs=+-  SaturateOnIntegerOverflow=on  InputSameDT=on  OutDataTypeStr=Inherit: Same as first input
  Sum3 : Sum  Inputs=2  SaturateOnIntegerOverflow=on  InputSameDT=on  OutDataTypeStr=Inherit: Same as first input
  "bool -> double" : DataTypeConversion  OutDataTypeStr=double  SaturateOnIntegerOverflow=on  RndMeth=Zero
  "bool -> double1" : DataTypeConversion  OutDataTypeStr=double  SaturateOnIntegerOverflow=on  RndMeth=Zero
  paf Fault : Subsystem
  sqrt1 : Math  Operator=sqrt  SaturateOnIntegerOverflow=on
  sqrt2 : Math  Operator=sqrt  SaturateOnIntegerOverflow=on
  m flow : Outport
  T flow : Outport  Port=2
  wires:
  "bool -> double1"/1 -> Sum3/2
  "bool -> double"/1 -> Sum/1
  Demux/3 -> T flow/1, H_in/2  "T upstream"
  Relational Operator1/1 -> "bool -> double1"/1
  Sign/1 -> H_in1/3  "Flow direction"
  Sum2/1 -> Sign/1
  Constant2/1 -> Sum3/1
  sqrt2/1 -> Multiport Switch2/2  "Non lineear region"
  Constant3/1 -> Relational Operator1/1, sqrt1/1
  sqrt1/1 -> H_lin2/1
  Sum1/1 -> sqrt2/1, Relational Operator1/2, H_lin2/2
  H_lin2/1 -> Multiport Switch2/3  "Linear region"
  H_in1/1 -> m flow/1
  Math Function/1 -> H_in1/2
  Multiport Switch2/1 -> H_in1/1
  Sum3/1 -> Multiport Switch2/1
  Relational Operator/1 -> "bool -> double"/1
  H_in/1 -> Math Function/1
  Demux/1 -> H_in/1, Sum1/1  "p upstream"
  Demux/2 -> Sum1/2  "p downstream"
  Multiport Switch1/1 -> Demux/1
  Mux1/1 -> Multiport Switch1/3
  Constant/1 -> Sum/2
  Sum/1 -> Multiport Switch1/1
  Mux/1 -> Multiport Switch1/2
  T down/1 -> Mux1/3
  T up/1 -> Mux/3
  p down/1 -> Relational Operator/2, Sum2/2, Mux1/1, Mux/2
  p up/1 -> Relational Operator/1, Sum2/1, Mux1/2, Mux/1
  Constant1/1 -> paf Fault/1(H)
  paf Fault/1(fpaf) -> H_in/3

== system Engine/Generic Single-Turbocharged Engine/Compressor ==
  p_af : Inport
  T_af : Inport  Port=2
  w_tc : Inport  Port=3
  T_ds : Inport  Port=4
  p_c : Inport  Port=5
  Compressor Example : Subsystem
  W_c : Outport
  T_c : Outport  Port=2
  Tq_c : Outport  Port=3
  wires:
  Compressor Example/1(W_c) -> W_c/1
  Compressor Example/2(T_c [K]) -> T_c/1
  p_c/1 -> Compressor Example/5(p_c [Pa])
  p_af/1 -> Compressor Example/1(p_af [Pa])
  Compressor Example/3(Tq_c [Nm]) -> Tq_c/1  "Tq_c"
  T_ds/1 -> Compressor Example/4(T_ds)
  w_tc/1 -> Compressor Example/3(w_tc [rad/s])
  T_af/1 -> Compressor Example/2(T_in [K])

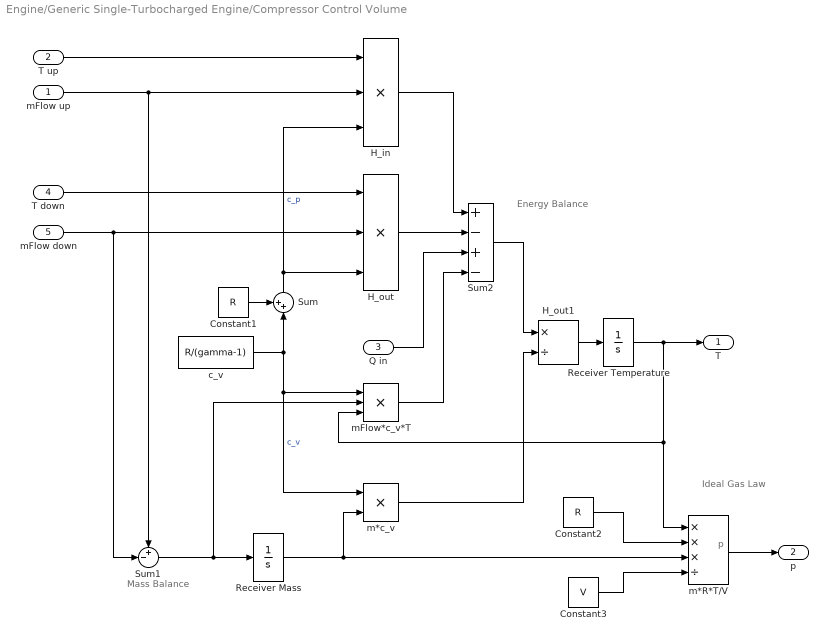
== system Engine/Generic Single-Turbocharged Engine/Compressor Control Volume ==
  note: Ideal Gas
      | Law
  note: Energy
      | Balance
  note: Mass
      | Balance
  note: p
  mFlow up : Inport
  T up : Inport  Port=2
  Q in : Inport  Port=3
  T down : Inport  Port=4
  mFlow down : Inport  Port=5
  Constant1 : Constant  Value=R
  Constant2 : Constant  Value=R
  Constant3 : Constant  Value=V
  H_in : Product  Inputs=3  SaturateOnIntegerOverflow=on  InputSameDT=on  OutDataTypeStr=Inherit: Same as first input
  H_out : Product  Inputs=3  SaturateOnIntegerOverflow=on  InputSameDT=on  OutDataTypeStr=Inherit: Same as first input
  H_out1 : Product  Inputs=*/  SaturateOnIntegerOverflow=on  InputSameDT=on  OutDataTypeStr=Inherit: Same as first input
  Receiver Mass : Integrator  InitialCondition=p_init*V/R/T_init  ZeroCross=off
  Receiver Temperature : Integrator  InitialCondition=T_init  ZeroCross=off
  Sum : Sum  Inputs=++|  SaturateOnIntegerOverflow=on  InputSameDT=on  OutDataTypeStr=Inherit: Same as first input
  Sum1 : Sum  Inputs=+-|  SaturateOnIntegerOverflow=on  InputSameDT=on  OutDataTypeStr=Inherit: Same as first input
  Sum2 : Sum  Inputs=+-+-  SaturateOnIntegerOverflow=on  InputSameDT=on  OutDataTypeStr=Inherit: Same as first input
  c_v : Constant  Value=R/(gamma-1)
  m*R*T/V : Product  Inputs=***/  SaturateOnIntegerOverflow=on  InputSameDT=on  OutDataTypeStr=Inherit: Same as first input
  m*c_v : Product  SaturateOnIntegerOverflow=on  InputSameDT=on  OutDataTypeStr=Inherit: Same as first input
  mFlow*c_v*T : Product  Inputs=3  SaturateOnIntegerOverflow=on  InputSameDT=on  OutDataTypeStr=Inherit: Same as first input
  T : Outport
  p : Outport  Port=2
  wires:
  mFlow*c_v*T/1 -> Sum2/4
  c_v/1 -> mFlow*c_v*T/1, m*c_v/1, Sum/2  "c_v"
  Sum1/1 -> mFlow*c_v*T/2, Receiver Mass/1
  Receiver Temperature/1 -> mFlow*c_v*T/3, m*R*T/V/1, T/1
  Constant2/1 -> m*R*T/V/2
  Constant3/1 -> m*R*T/V/4
  m*R*T/V/1 -> p/1
  H_out1/1 -> Receiver Temperature/1
  m*c_v/1 -> H_out1/2
  Sum2/1 -> H_out1/1
  Q in/1 -> Sum2/3
  H_out/1 -> Sum2/2
  H_in/1 -> Sum2/1
  mFlow up/1 -> Sum1/1, H_in/2
  mFlow down/1 -> H_out/2, Sum1/2
  T down/1 -> H_out/1
  T up/1 -> H_in/1
  Constant1/1 -> Sum/1
  Sum/1 -> H_out/3, H_in/3  "c_p"
  Receiver Mass/1 -> m*R*T/V/3, m*c_v/2

== system Engine/Generic Single-Turbocharged Engine/Engine ==
  p em : Inport
  w_e : Inport  Port=2
  T im : Inport  Port=3
  p im : Inport  Port=4
  lambda : Inport  Port=5
  AFs : Constant  Value=TC_ENGINE.fuel.AFs
  Engine Torque : Subsystem  mask(Engine Torque){V_d=TC_ENGINE.geometry.V_d, n_cyl=TC_ENGINE.geometry.n_cyl, bore=0.09, q_HV=44e6, AF_s=15.1, etaOtto=0.41, PI_bl=1.5, aux_dev=1.3, C_tq1=0.2e6, C_tq2=1.2e6}
      mask prompts: V_d "Displacement volume [m^3]"; n_cyl "Nymber of cylinders [-]"; bore "Bore [m]"; q_HV "Fuel lower heating value [J/kg]"; AF_s "Stoichiometric air to fuel ratio [-]"; etaOtto "Gross efficiency [-]"; PI_bl "Boost layout (>1) [-]"; aux_dev "Factor for auxilliary devices (>1) [-]"; C_tq1 "BMEP parameter C_tq1"; C_tq2 "BMEP parameter C_tq2"
      mask help:
      | Models the engine torque using:
      | 1) an ideal otto cycle model for the gross work produced by the combustion
      | 2) the ETH model for friction
      | 3) pumping work determined intake and exhaust manifold pressures
      mask Help:
      | Models the engine torque using:<br>
      | 1) an ideal otto cycle model for the gross work produced by the combustion<br>
      | 2) the ETH model for friction<br>
      | 3) pumping work determined intake and exhaust manifold pressures
  Engine flow : Subsystem  mask(Engine flow){V_d=TC_ENGINE.geometry.V_d, r_c=TC_ENGINE.geometry.r_c, C=0.8, R=TC_ENGINE.gasProp.air.R, K=TC_ENGINE.gasProp.exh.kappa}
      mask prompts: V_d "Engine displacement, V_d [m^3]"; r_c "Compression ratio, r_c [-]"; C "Volumetric constant, C [-]"; R "Ideal gas constant (fresh gas), R [J/kg K]"; K "Ratio of specific heats (exhaust  gamma) [-]"
      mask help:
      | The engine flow is modelled based on the volumetric efficiency. The volumetric efficiency is modelled using an ideal Otto cycle without valve overlap.
      |
      | mFlow=eta_vol*w_e*V_d*p_im/(4 pi R T_im)
      |
      | eta_vol=C*(r_c-(p_em/p_im)^(1/gamma))/(r_c-1)
      mask Help:
      | The engine flow is modelled based on the volumetric efficiency. The volumetric efficiency is modelled using an ideal Otto cycle without valve overlap.
      | <br>
      | mFlow=eta_vol*w_e*V_d*p_im/(4 pi R T_im)
      | <br>
      | eta_vol=C*(r_c-(p_em/p_im)^(1/gamma))/(r_c-1)
  Engine out temperature  (lambda=1) : Subsystem  mask(Engine out temperature){T_0=TC_ENGINE.exhTemp.zeroFlowTemp, C=TC_ENGINE.exhTemp.tempChangeWithFlow}
      mask prompts: T_0 "Zero flow temperature [K]"; C "Temperature change with flow [K s/kg]"
  Exhaust temperature drop Model 1 : Subsystem  mask(Exhaust heat transfer){corrSelector=Meisner Sorenson, D=TC_ENGINE.exhMan.eManDiam, L=TC_ENGINE.exhMan.eManLen, n_cyl=TC_ENGINE.exhMan.nrOfParallelPipes, h_ext=TC_ENGINE.exhMan.h_ext, R=TC_ENGINE.gasProp.exh.R, gamma=TC_ENGINE.gasProp.exh.kappa, mu=TC_ENGINE.exhMan.exh_mu, lambda=TC_ENGINE.exhMan.exh_lambda}
      mask prompts: corrSelector "Heat transfer correlation"; D "Pipe diameter [m]"; L "Pipe length [m]"; n_cyl "Number of parallell pipes [-]"; h_ext "External heat transfer coefficient [W/K m^2]"; R "Gas constant [J/kg K]"; gamma "Ratio of specific heats [-]"; mu "Dynamic viscosity (mu) [kg/m s]"; lambda "Thermal conductivity [W/m K]"
      mask help: Calculates the temperature drop in a pipe using the Model 1 in SAE paper by Lars Eriksson.
      mask Help: Calculates the temperature drop in a pipe using the Model 1 in SAE paper by Lars Eriksson.
      mask TypeOptions corrSelector: Meisner Sorenson | Shayler 1997a | Sieder Tate | Wendland Takedown | Wendland Tailpipe | Malcow et al | Caton Heywood | DOHC Downpipe | Valencia Downpipe | PROMEX | Woods | Blair | Standard | Standard Turbulent | Eriksson | Standard Laminar 2 | Reynolds
  Product : Product  Inputs=*//  SaturateOnIntegerOverflow=on  OutDataTypeStr=Inherit: Same as first input
  Saturation : Saturate  UpperLimit=350  LowerLimit=1  ZeroCross=off
  T_ambient1 : Constant  Value=TC_ENGINE.ambient.T
  To Workspace27 : ToWorkspace  VariableName=Tq_e_cb  SaveFormat=Timeseries  SampleTime=-1
  To Workspace28 : ToWorkspace  VariableName=Tq_e_f  SaveFormat=Timeseries  SampleTime=-1
  To Workspace29 : ToWorkspace  VariableName=Tq_e_p  SaveFormat=Timeseries  SampleTime=-1
  mFlow e : Outport
  T ti : Outport  Port=2
  Tq_e : Outport  Port=3
  air Flow : Outport  Port=4
  wires:
  Engine Torque/5(Pumping Torque) -> To Workspace29/1
  Engine out temperature  (lambda=1)/1(T out) -> Exhaust temperature drop Model 1/1(T in)
  Engine Torque/1(Net Torque) -> Saturation/1
  w_e/1 -> Engine Torque/1(omega engine), Engine flow/3(omega engine)
  p em/1 -> Engine Torque/4(p em), Engine flow/4(p em)
  p im/1 -> Engine Torque/3(p im), Engine flow/1(p im)
  Engine Torque/4(Friction torque) -> To Workspace28/1
  Engine Torque/3(Gross Torque) -> To Workspace27/1
  Product/1 -> Engine Torque/2(Fuel flow)
  Engine Torque/2(Exhaust mass flow) -> Exhaust temperature drop Model 1/2(mass flow), mFlow e/1, Engine out temperature  (lambda=1)/1(mass flow)
  T_ambient1/1 -> Exhaust temperature drop Model 1/3(T amb)
  Exhaust temperature drop Model 1/1(T out) -> T ti/1
  Engine flow/1(air mass flow) -> Engine Torque/5(Air Flow), air Flow/1, Product/1
  T im/1 -> Engine flow/2(T im)
  AFs/1 -> Product/2
  lambda/1 -> Product/3
  Saturation/1 -> Tq_e/1  "Tq_e [Nm]"

== system Engine/Generic Single-Turbocharged Engine/Exhaust Manifold Control Volume ==
  note: Ideal Gas
      | Law
  note: Energy
      | Balance
  note: Mass
      | Balance
  note: p
  mFlow up : Inport
  T up : Inport  Port=2
  Q in : Inport  Port=3
  T down : Inport  Port=4
  mFlow down : Inport  Port=5
  Constant1 : Constant  Value=R
  Constant2 : Constant  Value=R
  Constant3 : Constant  Value=V
  H_in : Product  Inputs=3  SaturateOnIntegerOverflow=on  InputSameDT=on  OutDataTypeStr=Inherit: Same as first input
  H_out : Product  Inputs=3  SaturateOnIntegerOverflow=on  InputSameDT=on  OutDataTypeStr=Inherit: Same as first input
  H_out1 : Product  Inputs=*/  SaturateOnIntegerOverflow=on  InputSameDT=on  OutDataTypeStr=Inherit: Same as first input
  Receiver Mass : Integrator  InitialCondition=p_init*V/R/T_init  ZeroCross=off
  Receiver Temperature : Integrator  InitialCondition=T_init  ZeroCross=off
  Sum : Sum  Inputs=++|  SaturateOnIntegerOverflow=on  InputSameDT=on  OutDataTypeStr=Inherit: Same as first input
  Sum1 : Sum  Inputs=+-|  SaturateOnIntegerOverflow=on  InputSameDT=on  OutDataTypeStr=Inherit: Same as first input
  Sum2 : Sum  Inputs=+-+-  SaturateOnIntegerOverflow=on  InputSameDT=on  OutDataTypeStr=Inherit: Same as first input
  c_v : Constant  Value=R/(gamma-1)
  m*R*T/V : Product  Inputs=***/  SaturateOnIntegerOverflow=on  InputSameDT=on  OutDataTypeStr=Inherit: Same as first input
  m*c_v : Product  SaturateOnIntegerOverflow=on  InputSameDT=on  OutDataTypeStr=Inherit: Same as first input
  mFlow*c_v*T : Product  Inputs=3  SaturateOnIntegerOverflow=on  InputSameDT=on  OutDataTypeStr=Inherit: Same as first input
  T : Outport
  p : Outport  Port=2
  wires:
  mFlow*c_v*T/1 -> Sum2/4
  c_v/1 -> mFlow*c_v*T/1, m*c_v/1, Sum/2  "c_v"
  Sum1/1 -> mFlow*c_v*T/2, Receiver Mass/1
  Receiver Temperature/1 -> mFlow*c_v*T/3, m*R*T/V/1, T/1
  Constant2/1 -> m*R*T/V/2
  Constant3/1 -> m*R*T/V/4
  m*R*T/V/1 -> p/1
  H_out1/1 -> Receiver Temperature/1
  m*c_v/1 -> H_out1/2
  Sum2/1 -> H_out1/1
  Q in/1 -> Sum2/3
  H_out/1 -> Sum2/2
  H_in/1 -> Sum2/1
  mFlow up/1 -> Sum1/1, H_in/2
  mFlow down/1 -> H_out/2, Sum1/2
  T down/1 -> H_out/1
  T up/1 -> H_in/1
  Constant1/1 -> Sum/1
  Sum/1 -> H_out/3, H_in/3  "c_p"
  Receiver Mass/1 -> m*R*T/V/3, m*c_v/2

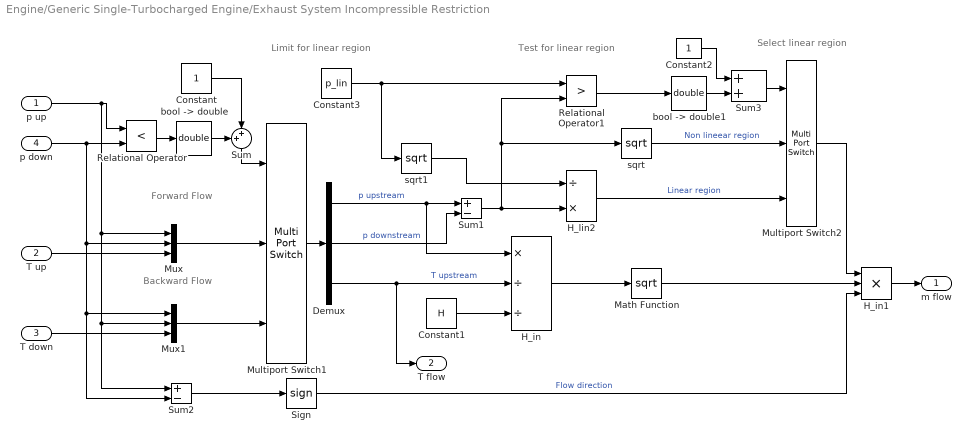
== system Engine/Generic Single-Turbocharged Engine/Exhaust System Incompressible Restriction ==
  note: Limit for linear region
  note: Select linear region
  note: Test for linear region
  note: Backward
      | Flow
  note: Forward
      | Flow
  p up : Inport
  T up : Inport  Port=2
  T down : Inport  Port=3
  p down : Inport  Port=4
  Constant : Constant
  Constant1 : Constant  Value=H
  Constant2 : Constant
  Constant3 : Constant  Value=p_lin
  Demux : Demux  Outputs=3
  H_in : Product  Inputs=*//  SaturateOnIntegerOverflow=on  InputSameDT=on  OutDataTypeStr=Inherit: Same as first input
  H_in1 : Product  Inputs=3  SaturateOnIntegerOverflow=on  InputSameDT=on  OutDataTypeStr=Inherit: Same as first input
  H_lin2 : Product  Inputs=/*  SaturateOnIntegerOverflow=on  InputSameDT=on  OutDataTypeStr=Inherit: Same as first input
  Math Function : Math  Operator=sqrt  SaturateOnIntegerOverflow=on
  Multiport Switch1 : MultiPortSwitch  Inputs=2  SaturateOnIntegerOverflow=on  InputSameDT=on
  Multiport Switch2 : MultiPortSwitch  Inputs=2  SaturateOnIntegerOverflow=on  InputSameDT=on
  Mux : Mux  Inputs=3
  Mux1 : Mux  Inputs=3
  Relational Operator : RelationalOperator  Operator=<  RndMeth=Nearest  InputSameDT=on
  Relational Operator1 : RelationalOperator  Operator=>  RndMeth=Nearest  InputSameDT=on
  Sign : Signum  ZeroCross=off
  Sum : Sum  Inputs=++|  SaturateOnIntegerOverflow=on  InputSameDT=on  OutDataTypeStr=Inherit: Same as first input
  Sum1 : Sum  Inputs=+-  SaturateOnIntegerOverflow=on  InputSameDT=on  OutDataTypeStr=Inherit: Same as first input
  Sum2 : Sum  Inputs=+-  SaturateOnIntegerOverflow=on  InputSameDT=on  OutDataTypeStr=Inherit: Same as first input
  Sum3 : Sum  Inputs=2  SaturateOnIntegerOverflow=on  InputSameDT=on  OutDataTypeStr=Inherit: Same as first input
  "bool -> double" : DataTypeConversion  OutDataTypeStr=double  SaturateOnIntegerOverflow=on  RndMeth=Zero
  "bool -> double1" : DataTypeConversion  OutDataTypeStr=double  SaturateOnIntegerOverflow=on  RndMeth=Zero
  sqrt : Math  Operator=sqrt  SaturateOnIntegerOverflow=on
  sqrt1 : Math  Operator=sqrt  SaturateOnIntegerOverflow=on
  m flow : Outport
  T flow : Outport  Port=2
  wires:
  "bool -> double1"/1 -> Sum3/2
  "bool -> double"/1 -> Sum/1
  Demux/3 -> T flow/1, H_in/2  "T upstream"
  Relational Operator1/1 -> "bool -> double1"/1
  Sign/1 -> H_in1/3  "Flow direction"
  Sum2/1 -> Sign/1
  Constant2/1 -> Sum3/1
  sqrt/1 -> Multiport Switch2/2  "Non lineear region"
  Constant3/1 -> Relational Operator1/1, sqrt1/1
  sqrt1/1 -> H_lin2/1
  Sum1/1 -> Relational Operator1/2, sqrt/1, H_lin2/2
  H_lin2/1 -> Multiport Switch2/3  "Linear region"
  H_in1/1 -> m flow/1
  Math Function/1 -> H_in1/2
  Multiport Switch2/1 -> H_in1/1
  Sum3/1 -> Multiport Switch2/1
  Relational Operator/1 -> "bool -> double"/1
  H_in/1 -> Math Function/1
  Constant1/1 -> H_in/3
  Demux/1 -> H_in/1, Sum1/1  "p upstream"
  Demux/2 -> Sum1/2  "p downstream"
  Multiport Switch1/1 -> Demux/1
  Mux1/1 -> Multiport Switch1/3
  Constant/1 -> Sum/2
  Sum/1 -> Multiport Switch1/1
  Mux/1 -> Multiport Switch1/2
  T down/1 -> Mux1/3
  T up/1 -> Mux/3
  p down/1 -> Relational Operator/2, Sum2/2, Mux1/1, Mux/2
  p up/1 -> Relational Operator/1, Sum2/1, Mux1/2, Mux/1

== system Engine/Generic Single-Turbocharged Engine/Inertia with friction ==
  note: inertia
  Tq_braking : Inport
  Tq_driving : Inport  Port=2
  Friction : Gain  Gain=w_friction  SaturateOnIntegerOverflow=on  OutDataTypeStr=Inherit: Same as input  ParamDataTypeStr=Inherit: Same as input
  Sum : Sum  Inputs=-+-  SaturateOnIntegerOverflow=on  InputSameDT=on  OutDataTypeStr=Inherit: Same as first input
  gain : Gain  Gain=1/Theta  SaturateOnIntegerOverflow=on  OutDataTypeStr=Inherit: Same as input  ParamDataTypeStr=Inherit: Same as input
  w_tc_IC : Integrator  InitialCondition=w_IC  LimitOutput=on  UpperSaturationLimit=w_upper  LowerSaturationLimit=w_lower  AbsoluteTolerance=1  ZeroCross=off
  w_tc : Outport
  wires:
  w_tc_IC/1 -> w_tc/1, Friction/1  "w_tc"
  Tq_braking/1 -> Sum/1
  Tq_driving/1 -> Sum/2
  gain/1 -> w_tc_IC/1
  Sum/1 -> gain/1
  Friction/1 -> Sum/3

== system Engine/Generic Single-Turbocharged Engine/Intake Manifold Control Volume ==
  note: Ideal Gas
      | Law
  note: Energy
      | Balance
  note: Mass
      | Balance
  note: p
  mFlow up : Inport
  T up : Inport  Port=2
  Q in : Inport  Port=3
  T down : Inport  Port=4
  mFlow down : Inport  Port=5
  Constant1 : Constant  Value=R
  Constant2 : Constant  Value=R
  Constant3 : Constant  Value=V
  H_in : Product  Inputs=3  SaturateOnIntegerOverflow=on  InputSameDT=on  OutDataTypeStr=Inherit: Same as first input
  H_out : Product  Inputs=3  SaturateOnIntegerOverflow=on  InputSameDT=on  OutDataTypeStr=Inherit: Same as first input
  H_out1 : Product  Inputs=*/  SaturateOnIntegerOverflow=on  InputSameDT=on  OutDataTypeStr=Inherit: Same as first input
  Receiver Mass : Integrator  InitialCondition=p_init*V/R/T_init  ZeroCross=off
  Receiver Temperature : Integrator  InitialCondition=T_init  ZeroCross=off
  Sum : Sum  Inputs=++|  SaturateOnIntegerOverflow=on  InputSameDT=on  OutDataTypeStr=Inherit: Same as first input
  Sum1 : Sum  Inputs=+-|  SaturateOnIntegerOverflow=on  InputSameDT=on  OutDataTypeStr=Inherit: Same as first input
  Sum2 : Sum  Inputs=+-+-  SaturateOnIntegerOverflow=on  InputSameDT=on  OutDataTypeStr=Inherit: Same as first input
  c_v : Constant  Value=R/(gamma-1)
  m*R*T/V : Product  Inputs=***/  SaturateOnIntegerOverflow=on  InputSameDT=on  OutDataTypeStr=Inherit: Same as first input
  m*c_v : Product  SaturateOnIntegerOverflow=on  InputSameDT=on  OutDataTypeStr=Inherit: Same as first input
  mFlow*c_v*T : Product  Inputs=3  SaturateOnIntegerOverflow=on  InputSameDT=on  OutDataTypeStr=Inherit: Same as first input
  T : Outport
  p : Outport  Port=2
  wires:
  mFlow*c_v*T/1 -> Sum2/4
  c_v/1 -> mFlow*c_v*T/1, m*c_v/1, Sum/2  "c_v"
  Sum1/1 -> mFlow*c_v*T/2, Receiver Mass/1
  Receiver Temperature/1 -> mFlow*c_v*T/3, m*R*T/V/1, T/1
  Constant2/1 -> m*R*T/V/2
  Constant3/1 -> m*R*T/V/4
  m*R*T/V/1 -> p/1
  H_out1/1 -> Receiver Temperature/1
  m*c_v/1 -> H_out1/2
  Sum2/1 -> H_out1/1
  Q in/1 -> Sum2/3
  H_out/1 -> Sum2/2
  H_in/1 -> Sum2/1
  mFlow up/1 -> Sum1/1, H_in/2
  mFlow down/1 -> H_out/2, Sum1/2
  T down/1 -> H_out/1
  T up/1 -> H_in/1
  Constant1/1 -> Sum/1
  Sum/1 -> H_out/3, H_in/3  "c_p"
  Receiver Mass/1 -> m*R*T/V/3, m*c_v/2
